simulink model "Controle_V"  (R2014a)
settings: Solver=ode45  StartTime=0.0  StopTime=3  RelTol=1e-3
values from neighbouring files (symbols this model uses):
  k = place(a,b,P)    [Controle_Posicao.m]
  k2 = place(a,b,P)    [Controle_Posicao.m]
settings Model: Creator=unieerisantos  LastModifiedBy=unieerisantos

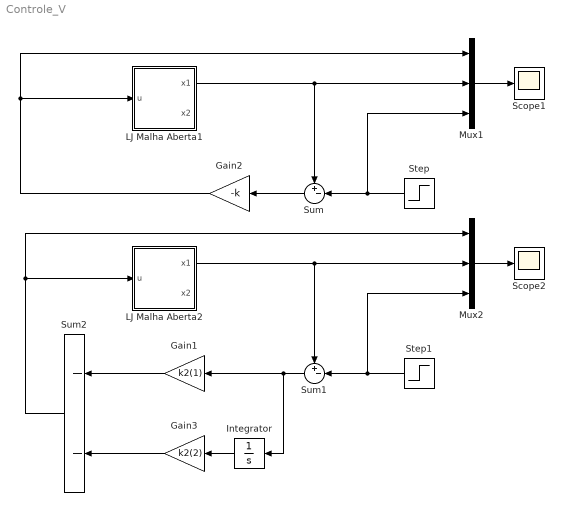
== system Controle_V ==
  Gain1 : Gain  Gain=k2(1)
  Gain2 : Gain  Gain=-k
  Gain3 : Gain  Gain=k2(2)
  Integrator : Integrator
  LJ Malha Aberta1 : Subsystem
  LJ Malha Aberta2 : Subsystem
  Mux1 : Mux  Inputs=3
  Mux2 : Mux  Inputs=3
  Scope1 : Scope
      settings: SaveName=ControleV
  Scope2 : Scope
  Step : Step  Time=0  After=10  SampleTime=0
  Step1 : Step  Time=0.5  After=10  SampleTime=0
  Sum : Sum  Inputs=+-|
  Sum1 : Sum  Inputs=+-|
  Sum2 : Sum  Inputs=--
  wires:
  LJ Malha Aberta1/1(x1) -> Sum/1, Mux1/2
  Gain2/1 -> Mux1/1, LJ Malha Aberta1/1(u)
  Mux1/1 -> Scope1/1
  Sum/1 -> Gain2/1
  Step/1 -> Sum/2, Mux1/3
  Mux2/1 -> Scope2/1
  Sum1/1 -> Integrator/1, Gain1/1
  Step1/1 -> Sum1/2, Mux2/3
  LJ Malha Aberta2/1(x1) -> Sum1/1, Mux2/2
  Gain3/1 -> Sum2/2
  Gain1/1 -> Sum2/1
  Integrator/1 -> Gain3/1
  Sum2/1 -> Mux2/1, LJ Malha Aberta2/1(u)

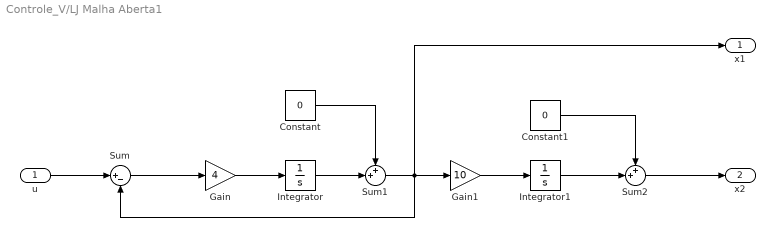
== system Controle_V/LJ Malha Aberta1 ==
  u : Inport
  Constant : Constant  Value=0
  Constant1 : Constant  Value=0
  Gain : Gain  Gain=4
  Gain1 : Gain  Gain=10
  Integrator : Integrator
  Integrator1 : Integrator
  Sum : Sum  Inputs=|+-
  Sum1 : Sum  Inputs=++|
  Sum2 : Sum  Inputs=++|
  x1 : Outport
  "x2 " : Outport  Port=2
  wires:
  Sum/1 -> Gain/1
  u/1 -> Sum/1
  Gain1/1 -> Integrator1/1
  Gain/1 -> Integrator/1
  Integrator/1 -> Sum1/2
  Sum1/1 -> Sum/2, x1/1, Gain1/1
  Constant/1 -> Sum1/1
  Integrator1/1 -> Sum2/2
  Constant1/1 -> Sum2/1
  Sum2/1 -> "x2 "/1

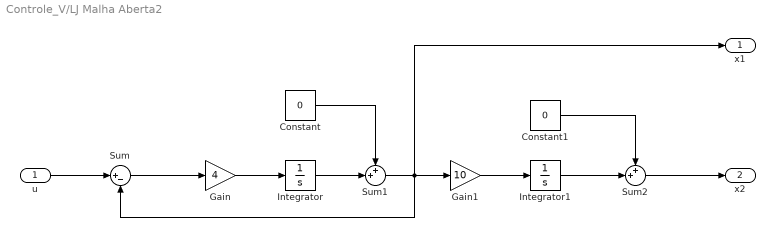
== system Controle_V/LJ Malha Aberta2 ==
  u : Inport
  Constant : Constant  Value=0
  Constant1 : Constant  Value=0
  Gain : Gain  Gain=4
  Gain1 : Gain  Gain=10
  Integrator : Integrator
  Integrator1 : Integrator
  Sum : Sum  Inputs=|+-
  Sum1 : Sum  Inputs=++|
  Sum2 : Sum  Inputs=++|
  x1 : Outport
  "x2 " : Outport  Port=2
  wires:
  Sum/1 -> Gain/1
  u/1 -> Sum/1
  Gain1/1 -> Integrator1/1
  Gain/1 -> Integrator/1
  Integrator/1 -> Sum1/2
  Sum1/1 -> Sum/2, x1/1, Gain1/1
  Constant/1 -> Sum1/1
  Integrator1/1 -> Sum2/2
  Constant1/1 -> Sum2/1
  Sum2/1 -> "x2 "/1
